simulink model "simpleTreeDiff"  (R2024b)
settings: Solver=VariableStepAuto  StartTime=0.0  StopTime=10.0  RelTol=1e-3
settings Model: Creator=neham  LastModifiedBy=neham

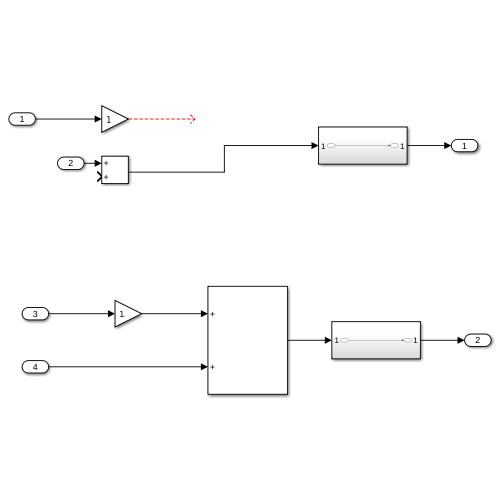
[thumbnail: Simulink's stored preview of the top-level diagram]
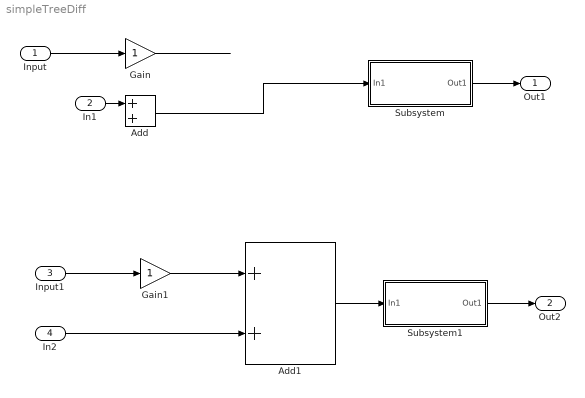
== system simpleTreeDiff ==
  Input : Inport
  In1 : Inport  Port=2
  Input1 : Inport  Port=3
  In2 : Inport  Port=4
  Add : Sum
  Add1 : Sum
  Gain : Gain
  Gain1 : Gain
  Subsystem : Subsystem
  Subsystem1 : Subsystem
  Out1 : Outport
  Out2 : Outport  Port=2
  wires:
  Input/1 -> Gain/1
  Gain/1 -> ?
  Add/1 -> Subsystem/1(In1)
  Subsystem/1(Out1) -> Out1/1
  Input1/1 -> Gain1/1
  Gain1/1 -> Add1/1
  Add1/1 -> Subsystem1/1(In1)
  In2/1 -> Add1/2
  Subsystem1/1(Out1) -> Out2/1
  In1/1 -> Add/1

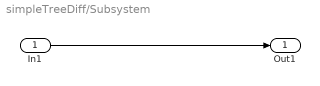
== system simpleTreeDiff/Subsystem ==
  In1 : Inport
  Out1 : Outport
  wires:
  In1/1 -> Out1/1

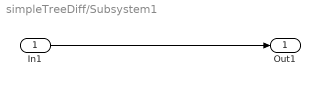
== system simpleTreeDiff/Subsystem1 ==
  In1 : Inport
  Out1 : Outport
  wires:
  In1/1 -> Out1/1
